simulink model "Subsystem"  (R2020a)
settings: Solver=FixedStepAuto  StartTime=0.0  StopTime=10.0  FixedStep=0.2  RelTol=1e-3
settings Model: Creator=I3  LastModifiedBy=I3
settings DataIOCC: SaveOutput=off  SaveTime=off

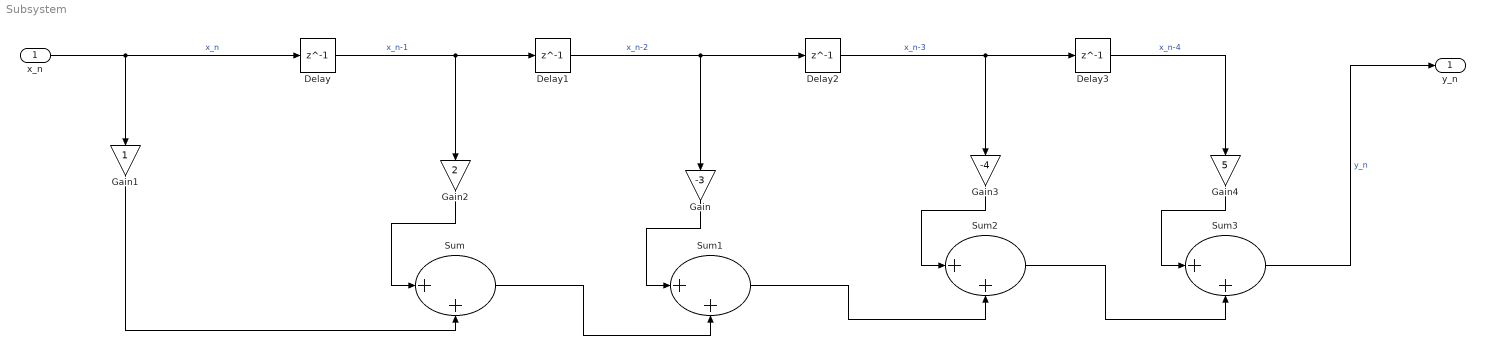
== system Subsystem ==
  x_n : Inport  OutDataTypeStr=double  PortDimensions=1  SampleTime=[0.20000000000000001,0]
  Delay{,1..3} (4 alike) : Delay  DelayLength=1  InitialCondition=0
  Gain : Gain  Gain=-3
  Gain1 : Gain
  Gain2 : Gain  Gain=2
  Gain3 : Gain  Gain=-4
  Gain4 : Gain  Gain=5
  Sum{,1..3} (4 alike) : Sum  Inputs=|++
  y_n : Outport  OutDataTypeStr=double  PortDimensions=1  SampleTime=[0.20000000000000001,0]
  wires:
  Delay1/1 -> Delay2/1, Gain/1  "x_n-2"
  Gain3/1 -> Sum2/1
  Delay/1 -> Gain2/1, Delay1/1  "x_n-1"
  Sum/1 -> Sum1/2
  x_n/1 -> Delay/1, Gain1/1  "x_n"
  Gain2/1 -> Sum/1
  Delay2/1 -> Delay3/1, Gain3/1  "x_n-3"
  Sum3/1 -> y_n/1  "y_n"
  Delay3/1 -> Gain4/1  "x_n-4"
  Gain1/1 -> Sum/2
  Gain/1 -> Sum1/1
  Sum1/1 -> Sum2/2
  Sum2/1 -> Sum3/2
  Gain4/1 -> Sum3/1
